simulink model "Brushless_DC_21"  (R2021b)
settings: Solver=VariableStepAuto  StartTime=0.0  StopTime=10.0  RelTol=1e-3
values from neighbouring files (symbols this model uses):
  J = 0.01    [param_pmsm.m]    (also in parameters_brushless_DC.m)
  k1phi = 5    [parameters_brushless_DC.m]
  L_A = 0.1    [parameters_brushless_DC.m]
  R_A = 5    [parameters_brushless_DC.m]
settings Model: Creator=student  LastModifiedBy=ganesh
settings DebuggingCC: UnconnectedInputMsg=none  UnconnectedOutputMsg=none  UnconnectedLineMsg=none
settings RTWCC: DLArmComputeVersion=20.02.1

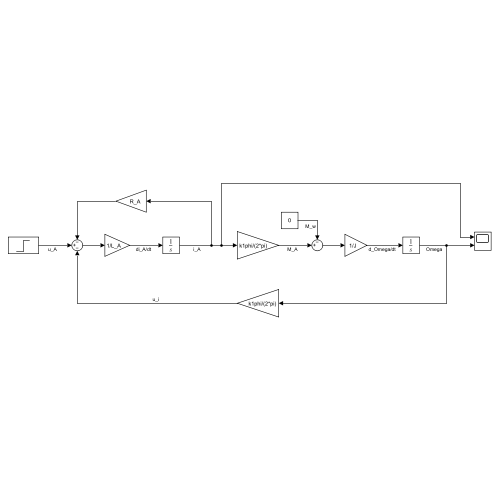
[thumbnail: Simulink's stored preview of the top-level diagram]
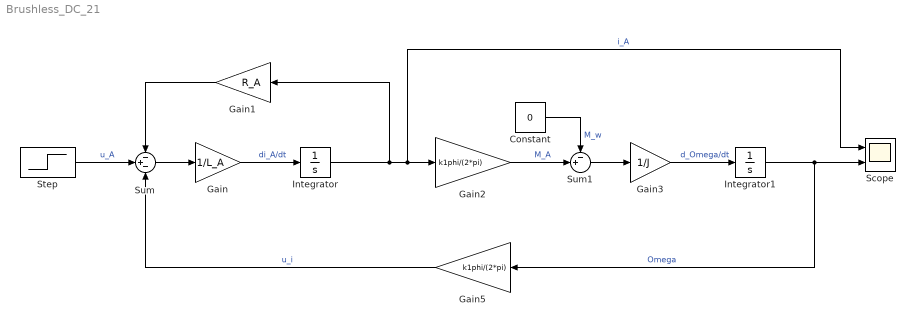
== system Brushless_DC_21 ==
  Constant : Constant  Value=0
  Gain : Gain  Gain=1/L_A
  Gain1 : Gain  Gain=R_A
  Gain2 : Gain  Gain=k1phi/(2*pi)
  Gain3 : Gain  Gain=1/J
  Gain5 : Gain  Gain=k1phi/(2*pi)
  Integrator : Integrator
  Integrator1 : Integrator
  Scope : Scope  NumInputPorts=2
  Step : Step  After=200  SampleTime=0
  Sum : Sum  Inputs=-+-
  Sum1 : Sum  Inputs=-+|
  wires:
  Gain/1 -> Integrator/1  "di_A/dt"
  Sum/1 -> Gain/1
  Step/1 -> Sum/2  "u_A"
  Integrator/1 -> Gain1/1, Scope/1, Gain2/1  "i_A"
  Gain1/1 -> Sum/1
  Gain2/1 -> Sum1/2  "M_A"
  Sum1/1 -> Gain3/1
  Gain3/1 -> Integrator1/1  "d_Omega/dt"
  Integrator1/1 -> Gain5/1, Scope/2  "Omega"
  Gain5/1 -> Sum/3  "u_i"
  Constant/1 -> Sum1/1  "M_w"
